simulink model "MATLAB_Exercise_5"  (R2017b)
settings: Solver=VariableStepAuto  StartTime=0.0  StopTime=5  RelTol=1e-3
settings Model: Creator=chenjiasheng  LastModifiedBy=chenjiasheng

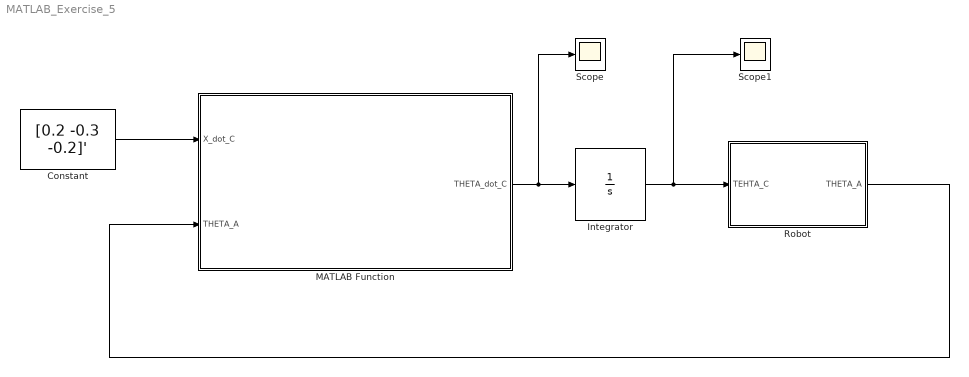
== system MATLAB_Exercise_5 ==
  Constant : Constant  Value=[0.2 -0.3 -0.2]'
  Integrator : Integrator  InitialCondition=[pi/18 pi/9 pi/6]'
  MATLAB Function : MATLAB Function  TreatAsAtomicUnit=on
  Robot : MATLAB Function  TreatAsAtomicUnit=on
  Scope : Scope
  Scope1 : Scope
  wires:
  Constant/1 -> MATLAB Function/1(X_dot_C)
  MATLAB Function/1(THETA_dot_C) -> Scope/1, Integrator/1
  Integrator/1 -> Scope1/1, Robot/1(TEHTA_C)
  Robot/1(THETA_A) -> MATLAB Function/2(THETA_A)

== matlab function MATLAB_Exercise_5/Robot ==
  data: TEHTA_C input; THETA_A output
function THETA_A = Robot(TEHTA_C)

THETA_A = TEHTA_C;
end

== matlab function MATLAB_Exercise_5/MATLAB Function ==
  data: X_dot_C input; THETA_dot_C output; THETA_A input
function THETA_dot_C = fcn(X_dot_C,THETA_A)
L1=4
L2=3
L3=2
theta1=THETA_A(1)
theta2=THETA_A(2)
theta3=THETA_A(3)
J=[-L1*sin(theta1)-L2*sin(theta1+theta2)-L3*sin(theta1+theta2+theta3) -L2*sin(theta1+theta2)-L3*sin(theta1+theta2+theta3) -L3*sin(theta1+theta2+theta3);
    L1*cos(theta1)+L2*cos(theta1+theta2)+L3*cos(theta1+theta2+theta3)  L2*cos(theta1+theta2)+L3*cos(theta1+theta2+theta3)  L3*cos(theta1+theta2+theta3);
    1                                                                  1                                                   1];

THETA_dot_C=inv(J)*X_dot_C
end
